simulink library "aero_librcs"  (R2021a)
settings: Solver=VariableStepAuto  StartTime=0.0  StopTime=10.0  RelTol=1e-3
values from neighbouring files (symbols this model uses):
  delt = .1    (= 0.1)    [aero_dap3dofdata.m]
libraries: aero_libdap x3
settings Model: RequirementInfo=9  ExtModeAutoUpdateStatusClock=off  Creator=The MathWorks, Inc.  LastModifiedBy=The MathWorks, Inc.
settings SolverCC: AlgebraicLoopSolver=TrustRegion
settings DataIOCC: SaveFormat=Array  SignalLoggingSaveFormat=ModelDataLogs  ReturnWorkspaceOutputs=off
settings OptimizationCC: BlockReduction=off  BooleanDataType=off
settings DebuggingCC: SaveWithParameterizedLinksMsg=none  SignalResolutionControl=TryResolveAllWithWarning  MultiTaskCondExecSysMsg=none  SFMachineParentedDataDiag=warning  ArithmeticOperatorsInVariantConditions=warning
settings HardwareCC: ProdBitPerPointer=32  ProdBitPerSizeT=32  ProdBitPerPtrDiffT=32  ProdLargestAtomicFloat=None  ProdIntDivRoundTo=Undefined  ProdEndianess=Unspecified  ProdWordSize=32  ProdHWDeviceType=32-bit Generic  TargetUnknown=on
settings ModelReferenceCC: PropagateSignalLabelsOutOfModel=off
settings SFSimCC: SimUseLocalCustomCode=off  CustomCodeUndefinedFunction=UseInterfaceOnly
settings RTWCC: RTWUseLocalCustomCode=off
settings ConfigComp: CovMetricSettings=d  CovSaveCumulativeToWorkspaceVar=on  CovSaveSingleToWorkspaceVar=on  CovExternalEMLEnable=off

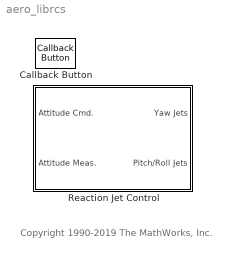
== system aero_librcs ==
  note: Copyright 1990-2019 The MathWorks, Inc.
  Callback Button : CallbackButton  ButtonText=?
      settings: ClickFcn=showExample('simulink_aerospace/DevelopingTheApolloLunarModuleDigitalAutopilotExample')
  Reaction Jet Control : Subsystem

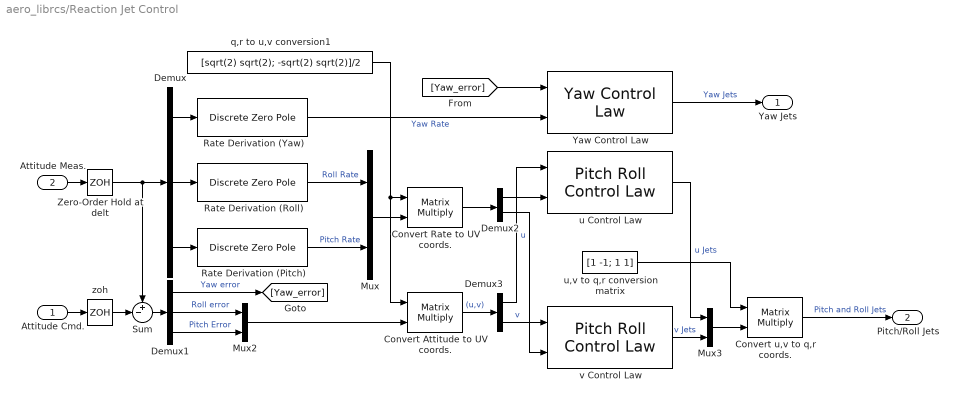
== system aero_librcs/Reaction Jet Control ==
  Attitude Cmd. : Inport  Unit=rad
  Attitude Meas. : Inport  Port=2  Unit=rad
  Convert Attitude to UV coords. : Product  Multiplication=Matrix(*)  InputSameDT=on  RndMeth=Zero  SaturateOnIntegerOverflow=on  OutDataTypeStr=Inherit: Same as first input
  Convert Rate to UV coords. : Product  Multiplication=Matrix(*)  InputSameDT=on  RndMeth=Zero  SaturateOnIntegerOverflow=on  OutDataTypeStr=Inherit: Same as first input
  Convert u,v to q,r coords. : Product  Multiplication=Matrix(*)  InputSameDT=on  RndMeth=Zero  SaturateOnIntegerOverflow=on  OutDataTypeStr=Inherit: Same as first input
  Demux : Demux  Outputs=3
      settings: DisplayOption=none
  Demux1 : Demux  Outputs=3
      settings: DisplayOption=none
  Demux2 : Demux  Outputs=2
      settings: DisplayOption=none
  Demux3 : Demux  Outputs=2
      settings: DisplayOption=none
  Mux : Mux  Inputs=2
  Mux2 : Mux  Inputs=2
  Mux3 : Mux  Inputs=2
  Rate Derivation (Pitch) : DiscreteZeroPole  Poles=[0]  Gain=1/delt  SampleTime=-1
  Rate Derivation (Roll) : DiscreteZeroPole  Poles=[0]  Gain=1/delt  SampleTime=-1
  Rate Derivation (Yaw) : DiscreteZeroPole  Poles=[0]  Gain=1/delt  SampleTime=-1
  Sum : Sum  Inputs=+-|  InputSameDT=on  SaturateOnIntegerOverflow=on  OutDataTypeStr=Inherit: Same as first input
  Yaw Control Law : aero_libdap/Yaw Control Law  alph=alph1  alphs=alphs1  DB=DB  tmin=tmin  delt=delt
      settings: SourceProductBaseCode=SL
  Zero-Order Hold at delt : ZeroOrderHold  SampleTime=delt
  q,r to u,v conversion1 : Constant  Value=[sqrt(2) sqrt(2); -sqrt(2) sqrt(2)]/2  VectorParams1D=off
  u Control Law : aero_libdap/Pitch Roll Control Law  alph=alphu  alphs=alphsu  DB=DB  tmin=tmin  delt=delt
      settings: SourceProductBaseCode=SL
  u,v to q,r conversion matrix : Constant  Value=[1 -1; 1 1]  VectorParams1D=off
  v Control Law : aero_libdap/Pitch Roll Control Law  alph=alphv  alphs=alphsv  DB=DB  tmin=tmin  delt=delt
      settings: SourceProductBaseCode=SL
  zoh : ZeroOrderHold  SampleTime=delt
  Yaw Jets : Outport  Unit=lbf  OutputWhenDisabled=reset  InitialOutput=0  VectorParamsAs1DForOutWhenUnconnected=off
  Pitch/Roll Jets : Outport  Port=2  Unit=lbf  OutputWhenDisabled=reset  InitialOutput=0  VectorParamsAs1DForOutWhenUnconnected=off
  wires:
  Demux3/1 -> u Control Law/1  "u"
  Convert u,v to q,r coords./1 -> Pitch/Roll Jets/1  "Pitch and Roll Jets"
  u,v to q,r conversion matrix/1 -> Convert u,v to q,r coords./1
  Mux3/1 -> Convert u,v to q,r coords./2
  Demux2/2 -> v Control Law/2
  Demux1/1 -> [Yaw_error]  "Yaw error"
  Demux2/1 -> u Control Law/2
  Demux3/2 -> v Control Law/1  "v"
  u Control Law/1 -> Mux3/1  "u Jets"
  v Control Law/1 -> Mux3/2  "v Jets"
  Attitude Cmd./1 -> zoh/1
  Mux2/1 -> Convert Attitude to UV coords./2
  Convert Attitude to UV coords./1 -> Demux3/1  "(u,v)"
  Convert Rate to UV coords./1 -> Demux2/1
  Demux1/3 -> Mux2/2  "Pitch Error"
  Demux1/2 -> Mux2/1  "Roll error"
  Sum/1 -> Demux1/1
  [Yaw_error] -> Yaw Control Law/1
  Yaw Control Law/1 -> Yaw Jets/1  "Yaw Jets"
  Rate Derivation (Yaw)/1 -> Yaw Control Law/2  "Yaw Rate"
  Attitude Meas./1 -> Zero-Order Hold at delt/1
  Mux/1 -> Convert Rate to UV coords./2
  Demux/1 -> Rate Derivation (Yaw)/1
  Demux/3 -> Rate Derivation (Pitch)/1
  Demux/2 -> Rate Derivation (Roll)/1
  Rate Derivation (Roll)/1 -> Mux/1  "Roll Rate"
  Rate Derivation (Pitch)/1 -> Mux/2  "Pitch Rate"
  q,r to u,v conversion1/1 -> Convert Rate to UV coords./1, Convert Attitude to UV coords./1
  Zero-Order Hold at delt/1 -> Demux/1, Sum/1
  zoh/1 -> Sum/2
